simulink model "Logan"  (R2024b)
settings: Solver=ode4  StartTime=0  StopTime=inf  FixedStep=0.01  RelTol=1e-3
values from neighbouring files (symbols this model uses):
  AltPoint = 100000    [Logan_init.m]
  area_secao = 79.402*1.5    (= 119.103)    [Logan_init.m]
  b = 9    [Logan_init.m]
  c = 15.252    [Logan_init.m]
  cp = 1003    [Logan_init.m]
  E = 110e9    (= 110000000000)    [Logan_init.m]
  eta_comb = 0.95    [Logan_init.m]
  Fuel_Freeze = 0    [Logan_init.m]
  g = 9.80665    [Logan_init.m]
  gamma = 1.4    [Logan_init.m]
  GammaRef_deg = 0    [Logan_init.m]
  h1 = 0.5746    [Logan_init.m]
  h2 = 0.7752    [Logan_init.m]
  h3 = 0.1502    [Logan_init.m]
  hc = h1 + h2 + h3    (= 1.5)    [Logan_init.m]
  he = 2.6    [Logan_init.m]
  Inertia = [Ixx 0 -Ixz; 0 Iyy 0; -Ixz 0 Izz]    [Logan_init.m]
  L = 22.5    [Logan_init.m]
  L_inlet = 5.5    [Logan_init.m]
  La = 5    [Logan_init.m]
  LHV = 120 * 10^6    (= 120000000)    [Logan_init.m]
  Ln0 = 4.8    [Logan_init.m]
  MachPoint = 10    [Logan_init.m]
  Manual_Control = 0    [Logan_init.m]
  MW_air = 28.85    [Logan_init.m]
  MW_H2 = 2.00    (= 2)    [Logan_init.m]
  PA_EngineMode = 0    [Logan_init.m]
  PA_LatMode = 2    [Logan_init.m]
  PA_LongMode = 2    [Logan_init.m]
  PA_TECSEngineInput = 0    [Logan_init.m]
  PhiPoint = 0    [Logan_init.m]
  R = 287    [Logan_init.m]
  RefMass_kg = 31000    [Logan_init.m]
  S = 91.5    [Logan_init.m]
  tau1 = 3.1    [Logan_init.m]
  tau2 = 18.23    [Logan_init.m]
  TECS_ON = 0    [Logan_init.m]
  theta1 = 4    [Logan_init.m]
  theta2 = 6    [Logan_init.m]
  theta_n = 4    [Logan_init.m]
  ThetaPoint = 0    [Logan_init.m]
  Trimming = 0    [Logan_init.m]    (also in Logan_trim.m)
  w = 3.000    (= 3)    [Logan_init.m]
  Waypoint_idx = 1    [Logan_init.m]
  Waypoints = [ ... (first row only)    [Logan_init.m]
  x_a = 3.7    [Logan_init.m]
  x_inlet = 6    [Logan_init.m]
  x_n0 = 3    [Logan_init.m]
  xf_m = 0    [Logan_init.m]
  y_cg = 0    [Logan_init.m]
  z_a = 0.4    [Logan_init.m]
  z_cg = -0.996    [Logan_init.m]
  z_inlet = 0.7    [Logan_init.m]
  zf_m = 0    [Logan_init.m]
undefined symbols (not defined in the file or in its folder): Earth, Receive, Send, WGS84
libraries: simulink x4, spsFirstOrderFilterLib x4, aerolibactuator x3, aerolibfltsims x2, aerolibatmos2 x1, aerolibtransform2 x1, aerolibanimutils x1, dspswit3 x1, spsEdgeDetectorLib x1
(part 2 of 5)

== system Logan/EqM/ExtForcesMoments ==
  LBE : Inport
  Mass_kg : Inport  Port=2
  GroundForcesMoments_N_Nm : Inport  Port=3
  AeroForcesMoments_N_Nm : Inport  Port=4
  ThrustForcesMoments_N_Nm : Inport  Port=5
  Add : Sum  Inputs=+++
  Constant : Constant  Value=0
  Demux : Demux  Outputs=2
  Demux1 : Demux  Outputs=3
  Divide : Product  Inputs=*/  Multiplication=Matrix(*)
  Gain : Gain  Gain=-1
  Math Function : Math  Operator=transpose  SignedPower=on
  Mux : Mux  Inputs=3
  Mux1 : Mux  Inputs=3
  Product : Product  Multiplication=Matrix(*)
  Sum : Sum  Inputs=|++
  g_mps2 : Gain  Gain=g
  ExtForces_N : Outport
  ExtMoments_Nm : Outport  Port=2
  LoadFactors : Outport  Port=3
  wires:
  Product/1 -> Sum/1  "Weight_N_body"
  Sum/1 -> ExtForces_N/1
  Divide/1 -> Demux1/1
  ThrustForcesMoments_N_Nm/1 -> Add/3
  Mux/1 -> Product/2
  Add/1 -> Demux/1
  LBE/1 -> Math Function/1
  g_mps2/1 -> Mux/3, Divide/2  "Weight_N"
  Mass_kg/1 -> g_mps2/1
  Demux1/1 -> Mux1/1  "nx"
  Demux1/2 -> Mux1/2  "ny"
  AeroForcesMoments_N_Nm/1 -> Add/2
  Mux1/1 -> LoadFactors/1
  Demux1/3 -> Gain/1
  Gain/1 -> Mux1/3  "nz"
  Demux/2 -> ExtMoments_Nm/1  "Moments"
  Constant/1 -> Mux/1, Mux/2
  GroundForcesMoments_N_Nm/1 -> Add/1
  Math Function/1 -> Product/1  "LEB"
  Demux/1 -> Divide/1, Sum/2  "Forces"

== system Logan/EqM/InertialData ==
  VB_mps : Inport
  LBE : Inport  Port=2
  Demux : Demux  Outputs=3
  Mux : Mux  Inputs=3
  Product : Product  Multiplication=Matrix(*)
  XI_m : Integrator  ContinuousStateAttributes='XI_m'
  YI_m1 : Integrator  ContinuousStateAttributes='YI_m'
  ZI_m : Integrator  ContinuousStateAttributes='ZI_m'
  PositionIntertial_m : Outport
  InertialVelocity_mps : Outport  Port=2
  wires:
  Demux/3 -> ZI_m/1
  Demux/2 -> YI_m1/1
  Demux/1 -> XI_m/1
  Product/1 -> Demux/1, InertialVelocity_mps/1  "VI_mps"
  ZI_m/1 -> Mux/3
  XI_m/1 -> Mux/1
  YI_m1/1 -> Mux/2
  Mux/1 -> PositionIntertial_m/1
  VB_mps/1 -> Product/2
  LBE/1 -> Product/1

== system Logan/EqM/TrajectoryData ==
  VI_mps : Inport
  Add : Sum
  Demux : Demux  Outputs=3
  Gain : Gain  Gain=-1
  Gain1 : Gain  Gain=180/pi
  Gain2 : Gain  Gain=180/pi
  Math Function : Math  Operator=square  SignedPower=on
  Math Function1 : Math  Operator=square  SignedPower=on
  Sqrt : Sqrt
  Trigonometric Function : Trigonometry  Operator=atan2
  Trigonometric Function1 : Trigonometry  Operator=atan2
  GroundSpeed_mps : Outport
  Gamma_deg : Outport  Port=2
  Track_deg : Outport  Port=3
  wires:
  VI_mps/1 -> Demux/1
  Trigonometric Function1/1 -> Gain2/1
  Gain/1 -> Trigonometric Function/1
  Add/1 -> Sqrt/1
  Demux/1 -> Math Function/1, Trigonometric Function1/2
  Sqrt/1 -> Trigonometric Function/2, GroundSpeed_mps/1
  Demux/2 -> Math Function1/1, Trigonometric Function1/1
  Demux/3 -> Gain/1
  Trigonometric Function/1 -> Gain1/1
  Math Function1/1 -> Add/2
  Math Function/1 -> Add/1
  Gain1/1 -> Gamma_deg/1
  Gain2/1 -> Track_deg/1

== system Logan/Inner Loop/EngineControl ==
  MachCmd : Inport
  Mach : Inport  Port=2
  Add7 : Sum  Inputs=+++
  Derivative1 : Derivative
  Gain21 : Gain  Gain=0.4
  Gain3 : Gain  Gain=8
  Gain6 : Gain  Gain=11
  Integrator3 : Integrator  LimitOutput=on  UpperSaturationLimit=10  LowerSaturationLimit=-1  ContinuousStateAttributes='Engine_MachInt'
  Sum18 : Sum  Inputs=|+-
  EngineCmd : Outport
  wires:
  MachCmd/1 -> Sum18/1
  Derivative1/1 -> Gain6/1
  Gain3/1 -> Add7/2
  Mach/1 -> Sum18/2
  Gain6/1 -> Add7/3
  Gain21/1 -> Add7/1
  Integrator3/1 -> Gain21/1
  Add7/1 -> EngineCmd/1
  Sum18/1 -> Derivative1/1, Gain3/1, Integrator3/1

== system Logan/Inner Loop/LateroDirectionalControl ==
  PhiCmd : Inport
  p_rps : Inport  Port=2
  r_rps : Inport  Port=3
  Beta_deg : Inport  Port=4
  Phi_deg : Inport  Port=5
  Add4 : Sum  Inputs=+++
  Add5 : Sum  Inputs=+++
  Beta_ref : Constant  Value=0
  Gain : Gain  Gain=-1.2
  Gain1 : Gain  Gain=pi/180
  Gain16 : Gain  Gain=0.3
  Gain17 : Gain  Gain=0.15
  Gain2 : Gain  Gain=-0.55
  Gain4 : Gain  Gain=-0.03
  Gain5 : Gain  Gain=-0.015
  Integrator : Integrator  ContinuousStateAttributes='Lat_PhiInt'
  Integrator1 : Integrator  ContinuousStateAttributes='Lat_BetaInt'
  Sum7 : Sum  Inputs=|+-
  Sum8 : Sum  Inputs=|+-
  AileronCmd : Outport
  RudderCmd : Outport  Port=2
  wires:
  Beta_deg/1 -> Sum8/2, Gain5/1  "Beta"
  Gain16/1 -> Add5/1
  Integrator1/1 -> Gain16/1
  Add5/1 -> RudderCmd/1
  Sum7/1 -> Gain1/1
  p_rps/1 -> Gain/1
  Add4/1 -> AileronCmd/1
  Gain17/1 -> Add4/1
  Integrator/1 -> Gain17/1
  Beta_ref/1 -> Sum8/1
  Gain5/1 -> Add5/2
  Gain2/1 -> Add5/3
  Gain4/1 -> Add4/2
  PhiCmd/1 -> Sum7/1
  r_rps/1 -> Gain2/1
  Phi_deg/1 -> Sum7/2, Gain4/1
  Sum8/1 -> Integrator1/1
  Gain1/1 -> Integrator/1
  Gain/1 -> Add4/3  "p_rps"

== system Logan/Inner Loop/LongitudinalControl ==
  Gamma_deg : Inport
  AlphaDot_rps : Inport  Port=2
  Q_Dyn_Pa : Inport  Port=3
  GammaCmd : Inport  Port=4
  Add6 : Sum  Inputs=+++
  GainScheduling1 : Subsystem
  GainScheduling2 : Subsystem
  GainScheduling3 : Subsystem
  Integrator2 : Integrator  LimitOutput=on  UpperSaturationLimit=8  LowerSaturationLimit=-8  ContinuousStateAttributes='Long_GammaInt'
  Sum16 : Sum  Inputs=|+-
  ElevCmd : Outport
  wires:
  Add6/1 -> ElevCmd/1
  GammaCmd/1 -> Sum16/1
  Gamma_deg/1 -> [Gamma_deg]
  [Gamma_deg] -> Sum16/2
  Sum16/1 -> Integrator2/1
  Q_Dyn_Pa/1 -> [Q_Dyn_Pa]
  [Q_Dyn_Pa] -> GainScheduling3/2(Q_Dyn_Pa)
  [Q_Dyn_Pa] -> GainScheduling1/2(Q_Dyn_Pa)
  [Q_Dyn_Pa] -> GainScheduling2/2(Q_Dyn_Pa)
  [Gamma_deg] -> GainScheduling1/1(Gamma_deg)
  GainScheduling1/1(Out1) -> Add6/1
  GainScheduling2/1(Out1) -> Add6/2
  Integrator2/1 -> GainScheduling2/1(GammaCmd)
  GainScheduling3/1(Out1) -> Add6/3
  AlphaDot_rps/1 -> GainScheduling3/1(AlphaDot_rps)

== system Logan/Inner Loop/Trimming ==
  ElevCmd : Inport
  Constant10 : Constant  Value=Trimming
  Constant9 : Constant  Value=0
  Switch : Switch  Criteria=u2 > Threshold  Threshold=0.5  SaturateOnIntegerOverflow=off  InputSameDT=off
  DeltaElevCmd : Outport
  wires:
  Constant9/1 -> Switch/1
  Constant10/1 -> Switch/2
  Switch/1 -> DeltaElevCmd/1
  ElevCmd/1 -> Switch/3

== system Logan/Inner Loop/Trimming1 ==
  AileronCmd : Inport
  Constant10 : Constant  Value=Trimming
  Constant9 : Constant  Value=0
  Switch : Switch  Criteria=u2 > Threshold  Threshold=0.5  SaturateOnIntegerOverflow=off  InputSameDT=off
  DeltaAileronCmd : Outport
  wires:
  Constant9/1 -> Switch/1
  Constant10/1 -> Switch/2
  Switch/1 -> DeltaAileronCmd/1
  AileronCmd/1 -> Switch/3

== system Logan/Inner Loop/Trimming2 ==
  RudderCmd : Inport
  Constant10 : Constant  Value=Trimming
  Constant9 : Constant  Value=0
  Switch : Switch  Criteria=u2 > Threshold  Threshold=0.5  SaturateOnIntegerOverflow=off  InputSameDT=off
  DeltaRudderCmd : Outport
  wires:
  Constant9/1 -> Switch/1
  Constant10/1 -> Switch/2
  Switch/1 -> DeltaRudderCmd/1
  RudderCmd/1 -> Switch/3

== system Logan/Inner Loop/Trimming3 ==
  EngineCmd : Inport
  Constant10 : Constant  Value=Trimming
  Constant9 : Constant  Value=0
  Switch : Switch  Criteria=u2 > Threshold  Threshold=0.5  SaturateOnIntegerOverflow=off  InputSameDT=off
  DeltaEngineCmd : Outport
  wires:
  Constant9/1 -> Switch/1
  Constant10/1 -> Switch/2
  Switch/1 -> DeltaEngineCmd/1
  EngineCmd/1 -> Switch/3

== system Logan/Mass Consumption/Fuel_Freeze ==
  1 : Inport
  Constant : Constant  Value=Fuel_Freeze
  Constant17 : Constant  Value=0
  Constant8 : Constant  Value=Trimming
  Logical Operator : Logic  Operator=OR  AllPortsSameDT=off  OutDataTypeStr=boolean
  Switch6 : Switch  Criteria=u2 > Threshold  Threshold=0.5  SaturateOnIntegerOverflow=off  InputSameDT=off
  2 : Outport
  wires:
  Constant17/1 -> Switch6/1
  1/1 -> Switch6/3
  Switch6/1 -> 2/1
  Logical Operator/1 -> Switch6/2
  Constant8/1 -> Logical Operator/1
  Constant/1 -> Logical Operator/2

== system Logan/Outer Loop/AltitudeMode ==
  Alt_ft : Inport
  Add8 : Sum
  AltPoint : Constant  Value=AltPoint
  Derivative2 : Derivative
  First-Order Filter3 : spsFirstOrderFilterLib/First-Order Filter  FilterType=Lowpass  Tc=0.5  Ts=0  Initialize=off  Vac_Init=[0, 0, 60]  Vdc_Init=0  PlotResponse=off  FreqRange="[0,  200,  1]"
  Gain11 : Gain  Gain=64e-5
  Gain12 : Gain  Gain=-128e-5
  Saturation7 : Saturate  UpperLimit=3  LowerLimit=-3
  Sum14 : Sum  Inputs=|+-
  Trimming1 : Subsystem
  AltRef : Outport
  wires:
  Gain12/1 -> Add8/2
  Alt_ft/1 -> Sum14/2, Derivative2/1
  Derivative2/1 -> Gain12/1
  Add8/1 -> Saturation7/1
  AltPoint/1 -> Sum14/1
  First-Order Filter3/1 -> Add8/1
  Sum14/1 -> Gain11/1
  Saturation7/1 -> AltRef/1
  Gain11/1 -> Trimming1/1(1)
  Trimming1/1(2) -> First-Order Filter3/1

== system Logan/Outer Loop/BankMode ==
  Phi_deg : Inport
  p_rps : Inport  Port=2
  Add8 : Sum  Inputs=+++
  Gain : Gain  Gain=1.2
  Gain11 : Gain  Gain=0.4
  Gain12 : Gain  Gain=1.2
  Integrator : Integrator
  PhiPoint : Constant  Value=PhiPoint
  Saturation : Saturate  UpperLimit=45  LowerLimit=-45
  Sum14 : Sum  Inputs=|+-
  Trimming1 : Subsystem
  PhiRef : Outport
  wires:
  Phi_deg/1 -> Sum14/2
  Add8/1 -> Saturation/1
  PhiPoint/1 -> Sum14/1
  Gain11/1 -> Add8/1
  p_rps/1 -> Gain12/1
  Saturation/1 -> PhiRef/1
  Sum14/1 -> Trimming1/1(1), Gain/1
  Integrator/1 -> Gain11/1
  Gain12/1 -> Add8/3
  Gain/1 -> Add8/2
  Trimming1/1(2) -> Integrator/1

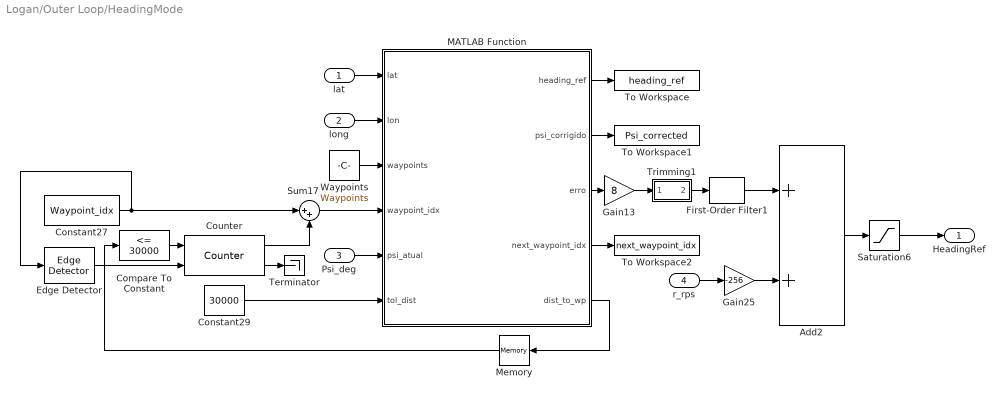
== system Logan/Outer Loop/HeadingMode ==
  lat : Inport
  long : Inport  Port=2
  Psi_deg : Inport  Port=3
  r_rps : Inport  Port=4
  Add2 : Sum
  Compare To Constant : simulink/Logic and Bit Operations/Compare To Constant  relop=<=  const=30000  OutDataTypeStr=boolean
  Constant27 : Constant  Value=Waypoint_idx  OutDataTypeStr=double
  Constant29 : Constant  Value=30000
  Counter : dspswit3/Counter  Direction=Up  CountEvent=Rising edge  CounterSize=User defined  MaxCount=255  InitialCount=0  Output=Count and Hit  HitValue=32  ResetInput=on  SamplesPerFrame=1  Ts=1  CntDtype=double  HitDtype=Logical
  Edge Detector : spsEdgeDetectorLib/Edge Detector  model=Either  ic=0  Ts=0
      settings: LibrarySourceBlock=sps_lib/Control/Edge Detector
  First-Order Filter1 : spsFirstOrderFilterLib/First-Order Filter  FilterType=Lowpass  Tc=10  Ts=0  Initialize=off  Vac_Init=[0, 0, 60]  Vdc_Init=0  PlotResponse=off  FreqRange="[0,  200,  1]"
  Gain13 : Gain  Gain=8
  Gain25 : Gain  Gain=-256
  MATLAB Function : MATLAB Function  TreatAsAtomicUnit=on
  Memory : Memory
  Saturation6 : Saturate  UpperLimit=75  LowerLimit=-75
  Sum17 : Sum  Inputs=|++
  Terminator : Terminator
  To Workspace : ToWorkspace  VariableName=heading_ref  SampleTime=-1
      settings: Save2DSignal=2-D array (concatenate along first dimension)
  To Workspace1 : ToWorkspace  VariableName=Psi_corrected  SampleTime=-1
      settings: Save2DSignal=2-D array (concatenate along first dimension)
  To Workspace2 : ToWorkspace  VariableName=next_waypoint_idx  SampleTime=-1
      settings: Save2DSignal=2-D array (concatenate along first dimension)
  Trimming1 : Subsystem
  Waypoints : Constant  Value=Waypoints  VectorParams1D=off
  HeadingRef : Outport
  wires:
  MATLAB Function/3(erro) -> Gain13/1
  MATLAB Function/4(next_waypoint_idx) -> To Workspace2/1
  Constant27/1 -> Edge Detector/1, Sum17/1
  Compare To Constant/1 -> Counter/1
  MATLAB Function/1(heading_ref) -> To Workspace/1
  Saturation6/1 -> HeadingRef/1
  Edge Detector/1 -> Counter/2
  Psi_deg/1 -> MATLAB Function/5(psi_atual)
  MATLAB Function/5(dist_to_wp) -> Memory/1
  long/1 -> MATLAB Function/2(lon)
  Sum17/1 -> MATLAB Function/4(waypoint_idx)
  MATLAB Function/2(psi_corrigido) -> To Workspace1/1
  Counter/2 -> Terminator/1
  Counter/1 -> Sum17/2
  Constant29/1 -> MATLAB Function/6(tol_dist)
  Memory/1 -> Compare To Constant/1
  lat/1 -> MATLAB Function/1(lat)
  First-Order Filter1/1 -> Add2/1
  Waypoints/1 -> MATLAB Function/3(waypoints)
  Gain25/1 -> Add2/2
  r_rps/1 -> Gain25/1
  Add2/1 -> Saturation6/1
  Gain13/1 -> Trimming1/1(1)
  Trimming1/1(2) -> First-Order Filter1/1

== system Logan/Outer Loop/MachMode ==
  MachPoint : Constant  Value=MachPoint
  Saturation : Saturate  UpperLimit=10  LowerLimit=5
  MachRef : Outport
  wires:
  MachPoint/1 -> Saturation/1
  Saturation/1 -> MachRef/1

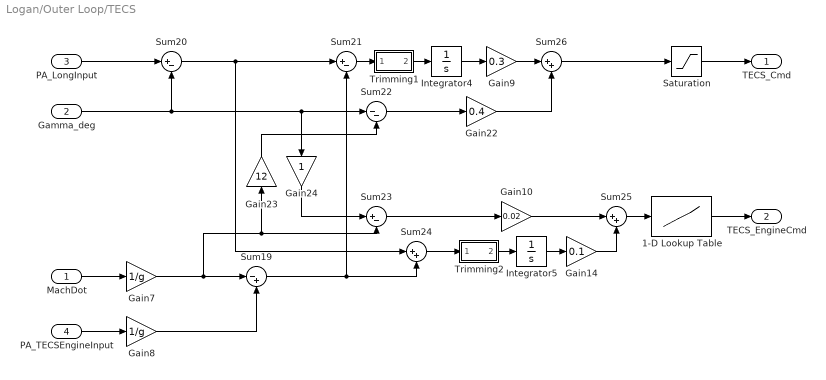
== system Logan/Outer Loop/TECS ==
  MachDot : Inport
  Gamma_deg : Inport  Port=2
  PA_LongInput : Inport  Port=3
  PA_TECSEngineInput : Inport  Port=4
  1-D Lookup Table : Lookup_n-D  NumberOfTableDimensions=1  BreakpointsForDimension1=[-5;-4;-3;-2;-1;0;1;2;3;4;5]  Table=[-1;-0.80000000000000004;-0.59999999999999998;-0.40000000000000002;-0.20000000000000001;0;0.20000000000000001;0.40000000000000002;0.59999999999999998;0.80000000000000004;1]  InternalRulePriority=Speed  RndMeth=Simplest
  Gain10 : Gain  Gain=0.02
  Gain14 : Gain  Gain=0.1
  Gain22 : Gain  Gain=0.4
  Gain23 : Gain  Gain=12
  Gain24 : Gain
  Gain7 : Gain  Gain=1/g
  Gain8 : Gain  Gain=1/g
  Gain9 : Gain  Gain=0.3
  Integrator4 : Integrator  UpperSaturationLimit=10  LowerSaturationLimit=-10
  Integrator5 : Integrator
  Saturation : Saturate  UpperLimit=3  LowerLimit=-3
  Sum19 : Sum  Inputs=|-+
  Sum20 : Sum  Inputs=|+-
  Sum21 : Sum  Inputs=|+-
  Sum22 : Sum  Inputs=|--
  Sum23 : Sum  Inputs=|+-
  Sum24 : Sum  Inputs=|++
  Sum25 : Sum  Inputs=|++
  Sum26 : Sum  Inputs=|++
  Trimming1 : Subsystem
  Trimming2 : Subsystem
  TECS_Cmd : Outport
  TECS_EngineCmd : Outport  Port=2
  wires:
  1-D Lookup Table/1 -> TECS_EngineCmd/1
  Sum23/1 -> Gain10/1
  Gamma_deg/1 -> Sum22/1, Gain24/1, Sum20/2
  Sum19/1 -> Sum21/2, Sum24/2
  Gain22/1 -> Sum26/2
  Sum22/1 -> Gain22/1
  PA_TECSEngineInput/1 -> Gain8/1
  Sum20/1 -> Sum21/1, Sum24/1
  Sum25/1 -> 1-D Lookup Table/1
  Gain7/1 -> Sum23/2, Gain23/1, Sum19/1
  Sum24/1 -> Trimming2/1(1)
  Gain23/1 -> Sum22/2
  Gain8/1 -> Sum19/2
  Gain10/1 -> Sum25/1
  Integrator5/1 -> Gain14/1
  Gain24/1 -> Sum23/1
  Integrator4/1 -> Gain9/1
  Gain9/1 -> Sum26/1
  Gain14/1 -> Sum25/2
  MachDot/1 -> Gain7/1
  PA_LongInput/1 -> Sum20/1
  Sum21/1 -> Trimming1/1(1)
  Trimming1/1(2) -> Integrator4/1
  Trimming2/1(2) -> Integrator5/1
  Sum26/1 -> Saturation/1
  Saturation/1 -> TECS_Cmd/1

== system Logan/Outer Loop/ThetaMode ==
  Theta_deg : Inport
  q_rps : Inport  Port=2
  Add8 : Sum  Inputs=+++
  Gain : Gain  Gain=1.4
  Gain11 : Gain  Gain=0.4
  Gain12 : Gain  Gain=0.6
  Integrator : Integrator
  Saturation : Saturate  UpperLimit=10  LowerLimit=-10
  Sum14 : Sum  Inputs=|+-
  ThetaPoint : Constant  Value=ThetaPoint
  Trimming1 : Subsystem
  ThetaRef : Outport
  wires:
  Theta_deg/1 -> Sum14/2
  Add8/1 -> Saturation/1
  ThetaPoint/1 -> Sum14/1
  q_rps/1 -> Gain12/1
  Gain11/1 -> Add8/1
  Saturation/1 -> ThetaRef/1
  Integrator/1 -> Gain11/1
  Gain12/1 -> Add8/3
  Gain/1 -> Add8/2
  Sum14/1 -> Trimming1/1(1)
  Trimming1/1(2) -> Gain/1, Integrator/1

== system Logan/Outer Loop/Trimming ==
  HeadingRef : Inport
  Constant22 : Constant  Value=0
  Constant23 : Constant  Value=Trimming
  Switch7 : Switch  Criteria=u2 > Threshold  Threshold=0.5  SaturateOnIntegerOverflow=off  InputSameDT=off
  PA_HeadingRef : Outport
  wires:
  Constant23/1 -> Switch7/2
  Constant22/1 -> Switch7/1
  Switch7/1 -> PA_HeadingRef/1
  HeadingRef/1 -> Switch7/3

== system Logan/Outer Loop/Trimming1 ==
  ThetaRef : Inport
  Constant17 : Constant  Value=0
  Constant8 : Constant  Value=Trimming
  Switch6 : Switch  Criteria=u2 > Threshold  Threshold=0.5  SaturateOnIntegerOverflow=off  InputSameDT=off
  PA_ThetaRef : Outport
  wires:
  Constant8/1 -> Switch6/2
  Constant17/1 -> Switch6/1
  ThetaRef/1 -> Switch6/3
  Switch6/1 -> PA_ThetaRef/1

== system Logan/Outer Loop/Trimming2 ==
  AltRef : Inport
  Constant17 : Constant  Value=0
  Constant8 : Constant  Value=Trimming
  Switch6 : Switch  Criteria=u2 > Threshold  Threshold=0.5  SaturateOnIntegerOverflow=off  InputSameDT=off
  PA_AltRef : Outport
  wires:
  Constant8/1 -> Switch6/2
  Constant17/1 -> Switch6/1
  AltRef/1 -> Switch6/3
  Switch6/1 -> PA_AltRef/1

== system Logan/Outer Loop/Trimming3 ==
  PhiRef : Inport
  Constant17 : Constant  Value=0
  Constant8 : Constant  Value=Trimming
  Switch6 : Switch  Criteria=u2 > Threshold  Threshold=0.5  SaturateOnIntegerOverflow=off  InputSameDT=off
  PA_PhiRef : Outport
  wires:
  Constant8/1 -> Switch6/2
  Constant17/1 -> Switch6/1
  PhiRef/1 -> Switch6/3
  Switch6/1 -> PA_PhiRef/1

== system Logan/Outer Loop/Trimming4 ==
  MachRef : Inport
  Constant17 : Constant  Value=0
  Constant8 : Constant  Value=Trimming
  Switch6 : Switch  Criteria=u2 > Threshold  Threshold=0.5  SaturateOnIntegerOverflow=off  InputSameDT=off
  PA_EngineCmd : Outport
  wires:
  Constant8/1 -> Switch6/2
  Constant17/1 -> Switch6/1
  MachRef/1 -> Switch6/3
  Switch6/1 -> PA_EngineCmd/1

== system Logan/Outer Loop/Trimming5 ==
  TECS : Inport
  Constant17 : Constant  Value=0
  Constant8 : Constant  Value=Trimming
  Switch6 : Switch  Criteria=u2 > Threshold  Threshold=0.5  SaturateOnIntegerOverflow=off  InputSameDT=off
  TECS_EngineCmd : Outport
  wires:
  Constant8/1 -> Switch6/2
  Constant17/1 -> Switch6/1
  TECS/1 -> Switch6/3
  Switch6/1 -> TECS_EngineCmd/1

== system Logan/Outer Loop/Trimming6 ==
  TECS : Inport
  Constant17 : Constant  Value=0
  Constant8 : Constant  Value=Trimming
  Switch6 : Switch  Criteria=u2 > Threshold  Threshold=0.5  SaturateOnIntegerOverflow=off  InputSameDT=off
  TECS_Cmd : Outport
  wires:
  Constant8/1 -> Switch6/2
  Constant17/1 -> Switch6/1
  TECS/1 -> Switch6/3
  Switch6/1 -> TECS_Cmd/1

== system Logan/Propulsion/EngineDynamics ==
  Thrust : Inport
  Filter_init : Subsystem
  First-Order Filter : spsFirstOrderFilterLib/First-Order Filter  FilterType=Lowpass  Tc=0.5  Ts=0  Initialize=off  Vac_Init=[0, 0, 60]  Vdc_Init=0  PlotResponse=off  FreqRange="[0,  200,  1]"
  Trimming : Subsystem
  T_thrust : Outport
  wires:
  Thrust/1 -> Trimming/2(Thrust), Filter_init/1(1)
  Trimming/1(T_Thrust) -> T_thrust/1
  First-Order Filter/1 -> Trimming/1(Thrust_Dyn)
  Filter_init/1(2) -> First-Order Filter/1

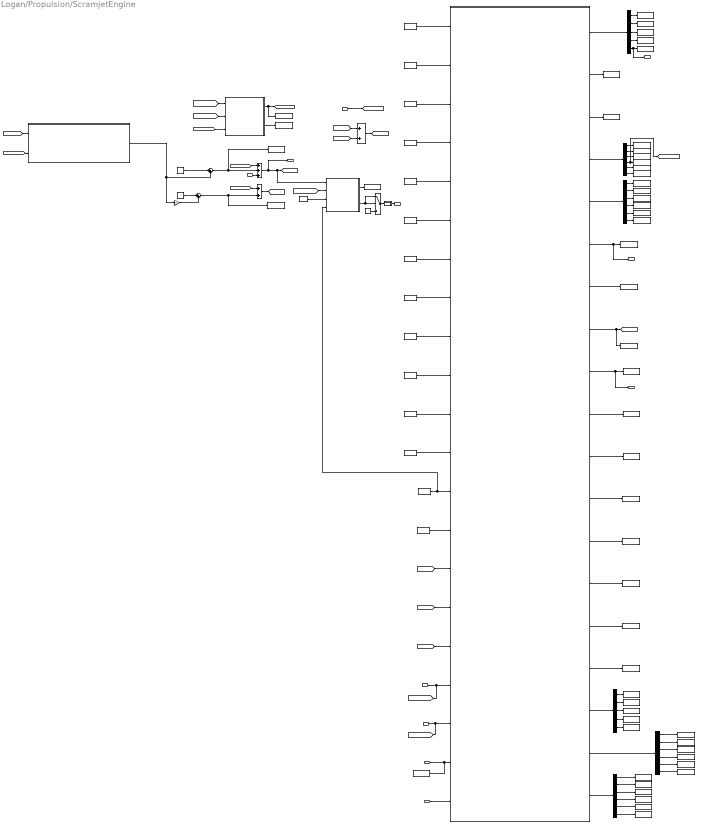
== system Logan/Propulsion/ScramjetEngine ==
  M1 : Inport
  T1 : Inport  Port=2
  p1 : Inport  Port=3
  Alpha : Inport  Port=4
  throttle : Inport  Port=5
  Delta_tau_f : Inport  Port=6
  Add : Sum  Inputs=+++
  Add1 : Sum
  Add2 : Sum
  Constant : Constant  Value=theta1
  Constant1 : Constant  Value=theta2
  Constant10 : Constant  Value=w
  Constant11 : Constant  Value=h1
  Constant12 : Constant  Value=h2
  Constant13 : Constant  Value=h3
  Constant14 : Constant  Value=hc
  Constant15 : Constant  Value=he
  Constant16 : Constant  Value=L_inlet
  Constant17 : Constant  Value=0
  Constant2 : Constant  Value=R
  Constant3 : Constant  Value=gamma
  Constant4 : Constant  Value=g
  Constant5 : Constant  Value=MW_H2
  Constant6 : Constant  Value=MW_air
  Constant7 : Constant  Value=LHV
  Constant8 : Constant  Value=eta_comb
  Constant9 : Constant  Value=cp
  Demux{,1,4..5} (4 alike) : Demux  Outputs=6
  Demux2 : Demux  Outputs=5
  Demux3 : Demux  Outputs=5
  Gain3 : Gain  Gain=2
  Ramp_Control : Subsystem
  Sum : Sum  Inputs=|++
  Sum1 : Sum  Inputs=|++
  Switch : Switch  Criteria=u2 > Threshold  SaturateOnIntegerOverflow=off  InputSameDT=off
  ThermodynamicModel : MATLAB Function  TreatAsAtomicUnit=on
  To Workspace : ToWorkspace  VariableName=m_dot_fuel  SampleTime=-1
      settings: Save2DSignal=2-D array (concatenate along first dimension)
  To Workspace1 : ToWorkspace  VariableName=M_ign  SampleTime=-1
      settings: Save2DSignal=2-D array (concatenate along first dimension)
  To Workspace10 : ToWorkspace  VariableName=M5  SampleTime=-1
      settings: Save2DSignal=2-D array (concatenate along first dimension)
  To Workspace11 : ToWorkspace  VariableName=M6  SampleTime=-1
      settings: Save2DSignal=2-D array (concatenate along first dimension)
  To Workspace12 : ToWorkspace  VariableName=M3  SampleTime=-1
      settings: Save2DSignal=2-D array (concatenate along first dimension)
  To Workspace13 : ToWorkspace  VariableName=ShockPoint  SampleTime=-1
      settings: Save2DSignal=2-D array (concatenate along first dimension)
  To Workspace14 : ToWorkspace  VariableName=T_ign  SampleTime=-1
      settings: Save2DSignal=2-D array (concatenate along first dimension)
  To Workspace15 : ToWorkspace  VariableName=p2  SampleTime=-1
      settings: Save2DSignal=2-D array (concatenate along first dimension)
  To Workspace16 : ToWorkspace  VariableName=p01  SampleTime=-1
      settings: Save2DSignal=2-D array (concatenate along first dimension)
  To Workspace17 : ToWorkspace  VariableName=T0  SampleTime=-1
      settings: Save2DSignal=2-D array (concatenate along first dimension)
  To Workspace18 : ToWorkspace  VariableName=p3  SampleTime=-1
      settings: Save2DSignal=2-D array (concatenate along first dimension)
  To Workspace19 : ToWorkspace  VariableName=p4  SampleTime=-1
      settings: Save2DSignal=2-D array (concatenate along first dimension)
  To Workspace2 : ToWorkspace  VariableName=T05_T0star_ratio  SampleTime=-1
      settings: Save2DSignal=2-D array (concatenate along first dimension)
  To Workspace20 : ToWorkspace  VariableName=p5  SampleTime=-1
      settings: Save2DSignal=2-D array (concatenate along first dimension)
  To Workspace21 : ToWorkspace  VariableName=p6  SampleTime=-1
      settings: Save2DSignal=2-D array (concatenate along first dimension)
  To Workspace22 : ToWorkspace  VariableName=T1  SampleTime=-1
      settings: Save2DSignal=2-D array (concatenate along first dimension)
  To Workspace23 : ToWorkspace  VariableName=fuel_air_ratio  SampleTime=-1
      settings: Save2DSignal=2-D array (concatenate along first dimension)
  To Workspace24 : ToWorkspace  VariableName=T2  SampleTime=-1
      settings: Save2DSignal=2-D array (concatenate along first dimension)
  To Workspace25 : ToWorkspace  VariableName=T3  SampleTime=-1
      settings: Save2DSignal=2-D array (concatenate along first dimension)
  To Workspace26 : ToWorkspace  VariableName=T4  SampleTime=-1
      settings: Save2DSignal=2-D array (concatenate along first dimension)
  To Workspace27 : ToWorkspace  VariableName=T5  SampleTime=-1
      settings: Save2DSignal=2-D array (concatenate along first dimension)
  To Workspace28 : ToWorkspace  VariableName=T6  SampleTime=-1
      settings: Save2DSignal=2-D array (concatenate along first dimension)
  To Workspace29 : ToWorkspace  VariableName=T_thrust  SampleTime=-1
      settings: Save2DSignal=2-D array (concatenate along first dimension)
  To Workspace3 : ToWorkspace  VariableName=q  SampleTime=-1
      settings: Save2DSignal=2-D array (concatenate along first dimension)
  To Workspace30 : ToWorkspace  VariableName=theta1_deg  SampleTime=-1
      settings: Save2DSignal=2-D array (concatenate along first dimension)
  To Workspace31 : ToWorkspace  VariableName=theta2_deg  SampleTime=-1
      settings: Save2DSignal=2-D array (concatenate along first dimension)
  To Workspace32 : ToWorkspace  VariableName=p1  SampleTime=-1
      settings: Save2DSignal=2-D array (concatenate along first dimension)
  To Workspace33 : ToWorkspace  VariableName=eta_t  SampleTime=-1
      settings: Save2DSignal=2-D array (concatenate along first dimension)
  To Workspace34 : ToWorkspace  VariableName=eta_prop  SampleTime=-1
      settings: Save2DSignal=2-D array (concatenate along first dimension)
  To Workspace35 : ToWorkspace  VariableName=q1  SampleTime=-1
      settings: Save2DSignal=2-D array (concatenate along first dimension)
  To Workspace36 : ToWorkspace  VariableName=eta_ex  SampleTime=-1
      settings: Save2DSignal=2-D array (concatenate along first dimension)
  To Workspace37 : ToWorkspace  VariableName=q2  SampleTime=-1
      settings: Save2DSignal=2-D array (concatenate along first dimension)
  To Workspace38 : ToWorkspace  VariableName=q3  SampleTime=-1
      settings: Save2DSignal=2-D array (concatenate along first dimension)
  To Workspace39 : ToWorkspace  VariableName=q4  SampleTime=-1
      settings: Save2DSignal=2-D array (concatenate along first dimension)
  To Workspace4 : ToWorkspace  VariableName=Inlet_drag  SampleTime=-1
      settings: Save2DSignal=2-D array (concatenate along first dimension)
  To Workspace40 : ToWorkspace  VariableName=q5  SampleTime=-1
      settings: Save2DSignal=2-D array (concatenate along first dimension)
  To Workspace41 : ToWorkspace  VariableName=eta_ex2  SampleTime=-1
      settings: Save2DSignal=2-D array (concatenate along first dimension)
  To Workspace42 : ToWorkspace  VariableName=eta_ex3  SampleTime=-1
      settings: Save2DSignal=2-D array (concatenate along first dimension)
  To Workspace43 : ToWorkspace  VariableName=eta_ex4  SampleTime=-1
      settings: Save2DSignal=2-D array (concatenate along first dimension)
  To Workspace44 : ToWorkspace  VariableName=eta_ex1  SampleTime=-1
      settings: Save2DSignal=2-D array (concatenate along first dimension)
  To Workspace45 : ToWorkspace  VariableName=eta_ex5  SampleTime=-1
      settings: Save2DSignal=2-D array (concatenate along first dimension)
  To Workspace46 : ToWorkspace  VariableName=eta_ex_total  SampleTime=-1
      settings: Save2DSignal=2-D array (concatenate along first dimension)
  To Workspace47 : ToWorkspace  VariableName=irre_total  SampleTime=-1
      settings: Save2DSignal=2-D array (concatenate along first dimension)
  To Workspace48 : ToWorkspace  VariableName=irre_stage2  SampleTime=-1
      settings: Save2DSignal=2-D array (concatenate along first dimension)
  To Workspace49 : ToWorkspace  VariableName=irre_stage3  SampleTime=-1
      settings: Save2DSignal=2-D array (concatenate along first dimension)
  To Workspace5 : ToWorkspace  VariableName=m_dot_air  SampleTime=-1
      settings: Save2DSignal=2-D array (concatenate along first dimension)
  To Workspace50 : ToWorkspace  VariableName=irre_stage1  SampleTime=-1
      settings: Save2DSignal=2-D array (concatenate along first dimension)
  To Workspace51 : ToWorkspace  VariableName=irre_stage4  SampleTime=-1
      settings: Save2DSignal=2-D array (concatenate along first dimension)
  To Workspace52 : ToWorkspace  VariableName=irre_stage5  SampleTime=-1
      settings: Save2DSignal=2-D array (concatenate along first dimension)
  To Workspace6 : ToWorkspace  VariableName=Isp  SampleTime=-1
      settings: Save2DSignal=2-D array (concatenate along first dimension)
  To Workspace7 : ToWorkspace  VariableName=M1  SampleTime=-1
      settings: Save2DSignal=2-D array (concatenate along first dimension)
  To Workspace8 : ToWorkspace  VariableName=M2  SampleTime=-1
      settings: Save2DSignal=2-D array (concatenate along first dimension)
  To Workspace9 : ToWorkspace  VariableName=M4  SampleTime=-1
      settings: Save2DSignal=2-D array (concatenate along first dimension)
  Trimming1 : Subsystem
  calculate_T3_M3 : MATLAB Function  TreatAsAtomicUnit=on
  calculate_shock_and_door : MATLAB Function  TreatAsAtomicUnit=on
  T_thrust : Outport
  p6 : Outport  Port=2
  door_length : Outport  Port=3
  m_dot_fuel : Outport  Port=4
  theta1_deg : Outport  Port=5
  wires:
  Add/1 -> theta1_deg/1, calculate_shock_and_door/1(theta1), [theta1_deg]
  Delta_tau_f/1 -> [delta_tau_f]
  [delta_tau_f] -> Add1/1
  ThermodynamicModel/6(T_thrust) -> To Workspace29/1, T_thrust/1
  Add1/1 -> [theta2_deg]
  [theta3_deg] -> ThermodynamicModel/17(theta3)
  Alpha/1 -> Add/3
  throttle/1 -> ThermodynamicModel/21(throttle)
  [theta1_deg] -> ThermodynamicModel/15(theta1)
  [theta2_deg] -> ThermodynamicModel/16(theta2)
  [delta_tau_f] -> Add/1
  [M1] -> calculate_T3_M3/2(M1)
  [T1] -> calculate_T3_M3/1(T1)
  ThermodynamicModel/8(f) -> To Workspace23/1, [f]
  [f] -> calculate_T3_M3/3(f)
  calculate_T3_M3/1(T3) -> To Workspace14/1, [T_ign]
  calculate_T3_M3/2(M3) -> To Workspace1/1
  ThermodynamicModel/4(temperatures) -> Demux/1
  ThermodynamicModel/5(mach_numbers) -> Demux1/1
  Demux/1 -> To Workspace22/1
  Demux/2 -> To Workspace24/1
  Demux/3 -> To Workspace25/1
  Demux/5 -> To Workspace27/1
  Demux/6 -> To Workspace28/1
  Demux1/1 -> To Workspace7/1
  Demux1/2 -> To Workspace8/1
  Demux1/3 -> To Workspace12/1
  Demux1/5 -> To Workspace10/1
  Demux1/6 -> To Workspace11/1
  Add2/1 -> [theta3_deg]
  [theta1_deg] -> Add2/1
  [theta2_deg] -> Add2/2
  Constant/1 -> Sum/1
  Constant1/1 -> Sum1/1
  [T_ign] -> Ramp_Control/1(T_Ign)
  [T4] -> Ramp_Control/2(T4)
  ThermodynamicModel/1(pressures) -> Demux2/1
  Demux2/1 -> To Workspace15/1
  Demux2/2 -> To Workspace18/1
  Demux2/5 -> To Workspace21/1, p6/1
  Demux2/4 -> To Workspace20/1
  Demux2/3 -> To Workspace19/1
  Sum1/1 -> Add1/2, To Workspace31/1
  Sum/1 -> To Workspace30/1, Add/2
  Gain3/1 -> Sum1/2
  ThermodynamicModel/9(m_dot_fuel) -> To Workspace/1, m_dot_fuel/1
  Constant2/1 -> ThermodynamicModel/1(R)
  Constant3/1 -> ThermodynamicModel/2(gamma)
  Constant4/1 -> ThermodynamicModel/3(g)
  Constant5/1 -> ThermodynamicModel/4(MW_H2)
  Constant6/1 -> ThermodynamicModel/5(MW_air)
  Constant7/1 -> ThermodynamicModel/6(LHV)
  Constant8/1 -> ThermodynamicModel/7(eta_comb)
  Constant9/1 -> ThermodynamicModel/8(cp)
  Constant10/1 -> ThermodynamicModel/9(w)
  Constant11/1 -> ThermodynamicModel/10(h1)
  Constant12/1 -> ThermodynamicModel/11(h2)
  Constant13/1 -> ThermodynamicModel/12(h3)
  Constant15/1 -> ThermodynamicModel/14(he)
  ThermodynamicModel/13(T05_T0star_ratio) -> To Workspace2/1
  ThermodynamicModel/12(q) -> To Workspace3/1
  ThermodynamicModel/11(D) -> To Workspace4/1
  ThermodynamicModel/10(m_dot_air) -> To Workspace5/1
  ThermodynamicModel/7(ISP) -> To Workspace6/1
  Demux1/4 -> To Workspace9/1
  [M1] -> calculate_shock_and_door/2(Mach)
  Constant16/1 -> calculate_shock_and_door/3(L_inlet)
  calculate_shock_and_door/1(ShockPoint) -> To Workspace13/1
  ThermodynamicModel/2(p01) -> To Workspace16/1
  ThermodynamicModel/3(T0) -> To Workspace17/1
  Demux/4 -> [T4], To Workspace26/1
  Switch/1 -> Trimming1/1(1)
  calculate_shock_and_door/2(door_length) -> Switch/1, Switch/2
  Constant17/1 -> Switch/3
  Trimming1/1(2) -> door_length/1
  Ramp_Control/1(DeltaTheta) -> Sum/2, Gain3/1
  ThermodynamicModel/14(eta_t) -> To Workspace33/1
  ThermodynamicModel/15(eta_prop) -> To Workspace34/1
  ThermodynamicModel/16(eta_ex) -> To Workspace36/1
  Demux3/4 -> To Workspace39/1
  Demux3/3 -> To Workspace38/1
  Demux3/1 -> To Workspace35/1
  Demux3/2 -> To Workspace37/1
  Demux3/5 -> To Workspace40/1
  ThermodynamicModel/17(Heat) -> Demux3/1
  Demux4/5 -> To Workspace45/1
  Demux4/3 -> To Workspace42/1
  Demux4/4 -> To Workspace43/1
  Demux4/2 -> To Workspace41/1
  Demux4/1 -> To Workspace44/1
  ThermodynamicModel/19(eta_stages) -> Demux4/1
  Demux4/6 -> To Workspace46/1
  Demux5/5 -> To Workspace52/1
  Demux5/6 -> To Workspace47/1
  Demux5/4 -> To Workspace51/1
  Demux5/3 -> To Workspace49/1
  Demux5/2 -> To Workspace48/1
  ThermodynamicModel/18(Irre) -> Demux5/1
  Demux5/1 -> To Workspace50/1
  p1/1 -> To Workspace32/1, ThermodynamicModel/20(p1)
  Constant14/1 -> calculate_shock_and_door/4(hc), ThermodynamicModel/13(hc)
  T1/1 -> [T1], ThermodynamicModel/19(T1)
  M1/1 -> [M1], ThermodynamicModel/18(M1)

== system Logan/EqM/BodyRates/CrossProduct ==
  A : Inport
  B : Inport  Port=2
  Add : Sum  Inputs=+-
  Demux : Demux  Outputs=3
  Demux1 : Demux  Outputs=3
  Mux : Mux  Inputs=3
  Mux1 : Mux  Inputs=3
  Product{,1..5} (6 alike) : Product
  C : Outport
  wires:
  Add/1 -> C/1  "A X B"
  Product2/1 -> Mux/3
  Product/1 -> Mux/1
  Demux/1 -> Product2/1, Product4/1
  Demux1/2 -> Product2/2, Product3/2
  Demux/3 -> Product1/1, Product3/1
  B/1 -> Demux1/1
  Mux1/1 -> Add/2
  Demux/2 -> Product/1, Product5/1
  A/1 -> Demux/1
  Product3/1 -> Mux1/1
  Demux1/1 -> Product1/2, Product5/2
  Mux/1 -> Add/1
  Product5/1 -> Mux1/3
  Product1/1 -> Mux/2
  Demux1/3 -> Product/2, Product4/2
  Product4/1 -> Mux1/2

== system Logan/EqM/BodyVelocities/CrossProduct ==
  A : Inport
  B : Inport  Port=2
  Add : Sum  Inputs=+-
  Demux : Demux  Outputs=3
  Demux1 : Demux  Outputs=3
  Mux : Mux  Inputs=3
  Mux1 : Mux  Inputs=3
  Product{,1..5} (6 alike) : Product
  C : Outport
  wires:
  Add/1 -> C/1  "A X B"
  Product2/1 -> Mux/3
  Product/1 -> Mux/1
  Demux/1 -> Product2/1, Product4/1
  Demux1/2 -> Product2/2, Product3/2
  Demux/3 -> Product1/1, Product3/1
  B/1 -> Demux1/1
  Mux1/1 -> Add/2
  Demux/2 -> Product/1, Product5/1
  A/1 -> Demux/1
  Product3/1 -> Mux1/1
  Demux1/1 -> Product1/2, Product5/2
  Mux/1 -> Add/1
  Product5/1 -> Mux1/3
  Product1/1 -> Mux/2
  Demux1/3 -> Product/2, Product4/2
  Product4/1 -> Mux1/2

== system Logan/EqM/EulerAngles/EulerRates ==
  BodyRates_radps : Inport
  EulerAngles_rad : Inport  Port=2
  Abs : Abs  SaturateOnIntegerOverflow=off
  Constant : Constant  Value=0.001
  Demux : Demux  Outputs=3
  Mux : Mux  Inputs=3
  Mux1 : Mux  Inputs=3
  Mux2 : Mux  Inputs=3
  Product : Product
  Relay : Relay  OnSwitchValue=.001  OffSwitchValue=0  OnOutputValue=0  OffOutputValue=1
  Sign : Signum
  Switch : Switch  Criteria=u2 > Threshold  Threshold=0.5  SaturateOnIntegerOverflow=off  InputSameDT=off
  Trigonometric Function : Trigonometry  Operator=sincos
  phidot_radps2 : Fcn  Expr=u(1)+u(2)*u(4)*(u(5)/u(8))+u(3)*u(7)*(u(5)/u(8))
  psidot_radps2 : Fcn  Expr=(u(2)*u(4)+u(3)*u(7))/u(8)
  thetadot_radps2 : Fcn  Expr=u(2)*u(7)-u(3)*u(4)
  EulerRates_radsps2 : Outport
  wires:
  Mux1/1 -> Mux/3
  Trigonometric Function/1 -> Mux/2
  Demux/3 -> Mux1/3
  Constant/1 -> Product/1
  Sign/1 -> Product/2
  Switch/1 -> Mux1/2
  Demux/2 -> Switch/3, Abs/1, Sign/1
  Mux2/1 -> EulerRates_radsps2/1
  psidot_radps2/1 -> Mux2/3
  Product/1 -> Switch/1
  Abs/1 -> Relay/1
  thetadot_radps2/1 -> Mux2/2
  phidot_radps2/1 -> Mux2/1
  BodyRates_radps/1 -> Mux/1
  Relay/1 -> Switch/2
  Demux/1 -> Mux1/1
  Trigonometric Function/2 -> Demux/1
  EulerAngles_rad/1 -> Trigonometric Function/1
  Mux/1 -> psidot_radps2/1, thetadot_radps2/1, phidot_radps2/1

== system Logan/EqM/EulerAngles/LBE_rotation ==
  note: LBE
  EulerAngles_rad : Inport
  Math Function : Math  Operator=transpose  SignedPower=on
  Mux : Mux  Inputs=2
  Mux2 : Mux  Inputs=9
  Reshape : Reshape  OutputDimensionality=Customize  OutputDimensions=[3,3]
  Trigonometric Function : Trigonometry  Operator=sincos
  phidot_radps1 : Fcn  Expr=u(1)*u(2)*u(6) - u(4)*u(3)
  phidot_radps2 : Fcn  Expr=u(5)*u(6)
  phidot_radps3 : Fcn  Expr=u(6)*u(2)*u(4) + u(1)*u(3)
  phidot_radps4 : Fcn  Expr=u(5)*u(3)
  phidot_radps5 : Fcn  Expr=u(1)*u(2)*u(3) + u(4)*u(6)
  phidot_radps6 : Fcn  Expr=u(4)*u(2)*u(3) -u(1)*u(6)
  phidot_radps7 : Fcn  Expr=-u(2)
  phidot_radps8 : Fcn  Expr=u(1)*u(5)
  phidot_radps9 : Fcn  Expr=u(4)*u(5)
  LBE : Outport
  wires:
  phidot_radps9/1 -> Mux2/9
  phidot_radps8/1 -> Mux2/8
  phidot_radps7/1 -> Mux2/7
  phidot_radps5/1 -> Mux2/5
  phidot_radps6/1 -> Mux2/6
  Mux/1 -> phidot_radps4/1, phidot_radps5/1, phidot_radps6/1, phidot_radps7/1, phidot_radps8/1, phidot_radps9/1, phidot_radps2/1, phidot_radps1/1, phidot_radps3/1
  Trigonometric Function/1 -> Mux/1
  phidot_radps1/1 -> Mux2/2
  phidot_radps2/1 -> Mux2/1
  phidot_radps4/1 -> Mux2/4
  phidot_radps3/1 -> Mux2/3
  Math Function/1 -> LBE/1
  Reshape/1 -> Math Function/1
  Mux2/1 -> Reshape/1
  Trigonometric Function/2 -> Mux/2
  EulerAngles_rad/1 -> Trigonometric Function/1

== system Logan/Inner Loop/LongitudinalControl/GainScheduling1 ==
  Gamma_deg : Inport
  Q_Dyn_Pa : Inport  Port=2
  2-D Lookup Table : Lookup_n-D  NumberOfTableDimensions=1  BreakpointsForDimension1=[83734; 1.70e5; 851500]  BreakpointsForDimension2=[1:3]  Table=[-40; -32; -32]  InternalRulePriority=Speed  RndMeth=Simplest
  Product : Product
  Saturation : Saturate  UpperLimit=-32  LowerLimit=-65
  Out1 : Outport
  wires:
  2-D Lookup Table/1 -> Saturation/1
  Q_Dyn_Pa/1 -> 2-D Lookup Table/1
  Gamma_deg/1 -> Product/1
  Product/1 -> Out1/1
  Saturation/1 -> Product/2

== system Logan/Inner Loop/LongitudinalControl/GainScheduling2 ==
  GammaCmd : Inport
  Q_Dyn_Pa : Inport  Port=2
  2-D Lookup Table : Lookup_n-D  NumberOfTableDimensions=1  BreakpointsForDimension1=[83734; 1.70e5; 851500]  BreakpointsForDimension2=[1:3]  Table=[12; 16;16]  InternalRulePriority=Speed  RndMeth=Simplest
  Product : Product
  Saturation : Saturate  UpperLimit=16  LowerLimit=3
  Out1 : Outport
  wires:
  2-D Lookup Table/1 -> Saturation/1
  Q_Dyn_Pa/1 -> 2-D Lookup Table/1
  GammaCmd/1 -> Product/1
  Product/1 -> Out1/1
  Saturation/1 -> Product/2

== system Logan/Inner Loop/LongitudinalControl/GainScheduling3 ==
  AlphaDot_rps : Inport
  Q_Dyn_Pa : Inport  Port=2
  2-D Lookup Table : Lookup_n-D  NumberOfTableDimensions=1  BreakpointsForDimension1=[83734; 1.70e5; 851500]  BreakpointsForDimension2=[1:3]  Table=[15; 32; 32]  InternalRulePriority=Speed  RndMeth=Simplest
  Product : Product
  Saturation : Saturate  UpperLimit=32  LowerLimit=19
  Out1 : Outport
  wires:
  2-D Lookup Table/1 -> Saturation/1
  Q_Dyn_Pa/1 -> 2-D Lookup Table/1
  AlphaDot_rps/1 -> Product/1
  Product/1 -> Out1/1
  Saturation/1 -> Product/2

== system Logan/Outer Loop/AltitudeMode/Trimming1 ==
  1 : Inport
  Constant17 : Constant  Value=0
  Constant8 : Constant  Value=Trimming
  Switch6 : Switch  Criteria=u2 > Threshold  Threshold=0.5  SaturateOnIntegerOverflow=off  InputSameDT=off
  2 : Outport
  wires:
  Constant8/1 -> Switch6/2
  Constant17/1 -> Switch6/1
  1/1 -> Switch6/3
  Switch6/1 -> 2/1

== system Logan/Outer Loop/BankMode/Trimming1 ==
  1 : Inport
  Constant17 : Constant  Value=0
  Constant8 : Constant  Value=Trimming
  Switch6 : Switch  Criteria=u2 > Threshold  Threshold=0.5  SaturateOnIntegerOverflow=off  InputSameDT=off
  2 : Outport
  wires:
  Constant8/1 -> Switch6/2
  Constant17/1 -> Switch6/1
  1/1 -> Switch6/3
  Switch6/1 -> 2/1

== system Logan/Outer Loop/HeadingMode/Trimming1 ==
  1 : Inport
  Constant17 : Constant  Value=0
  Constant8 : Constant  Value=Trimming
  Switch6 : Switch  Criteria=u2 > Threshold  Threshold=0.5  SaturateOnIntegerOverflow=off  InputSameDT=off
  2 : Outport
  wires:
  Constant8/1 -> Switch6/2
  Constant17/1 -> Switch6/1
  1/1 -> Switch6/3
  Switch6/1 -> 2/1

== system Logan/Outer Loop/TECS/Trimming1 ==
  1 : Inport
  Constant17 : Constant  Value=0
  Constant8 : Constant  Value=Trimming
  Switch6 : Switch  Criteria=u2 > Threshold  Threshold=0.5  SaturateOnIntegerOverflow=off  InputSameDT=off
  2 : Outport
  wires:
  Constant8/1 -> Switch6/2
  Constant17/1 -> Switch6/1
  1/1 -> Switch6/3
  Switch6/1 -> 2/1

== system Logan/Outer Loop/TECS/Trimming2 ==
  1 : Inport
  Constant17 : Constant  Value=0
  Constant8 : Constant  Value=Trimming
  Switch6 : Switch  Criteria=u2 > Threshold  Threshold=0.5  SaturateOnIntegerOverflow=off  InputSameDT=off
  2 : Outport
  wires:
  Constant8/1 -> Switch6/2
  Constant17/1 -> Switch6/1
  1/1 -> Switch6/3
  Switch6/1 -> 2/1

== system Logan/Outer Loop/ThetaMode/Trimming1 ==
  1 : Inport
  Constant17 : Constant  Value=0
  Constant8 : Constant  Value=Trimming
  Switch6 : Switch  Criteria=u2 > Threshold  Threshold=0.5  SaturateOnIntegerOverflow=off  InputSameDT=off
  2 : Outport
  wires:
  Constant8/1 -> Switch6/2
  Constant17/1 -> Switch6/1
  1/1 -> Switch6/3
  Switch6/1 -> 2/1

== system Logan/Propulsion/EngineDynamics/Filter_init ==
  1 : Inport
  Constant : Constant  Value=0
  Constant8 : Constant  Value=Trimming
  Switch6 : Switch  Criteria=u2 > Threshold  Threshold=0.5  SaturateOnIntegerOverflow=off  InputSameDT=off
  2 : Outport
  wires:
  Constant8/1 -> Switch6/2
  Switch6/1 -> 2/1
  1/1 -> Switch6/3
  Constant/1 -> Switch6/1

== system Logan/Propulsion/EngineDynamics/Trimming ==
  Thrust_Dyn : Inport
  Thrust : Inport  Port=2
  Constant8 : Constant  Value=Trimming
  Switch6 : Switch  Criteria=u2 > Threshold  Threshold=0.5  SaturateOnIntegerOverflow=off  InputSameDT=off
  T_Thrust : Outport
  wires:
  Constant8/1 -> Switch6/2
  Switch6/1 -> T_Thrust/1
  Thrust_Dyn/1 -> Switch6/3
  Thrust/1 -> Switch6/1

== system Logan/Propulsion/ScramjetEngine/Ramp_Control ==
  T_Ign : Inport
  T4 : Inport  Port=2
  Add3 : Sum  Inputs=3
  Derivative : Derivative
  First-Order Filter : spsFirstOrderFilterLib/First-Order Filter  FilterType=Lowpass  Tc=30  Ts=0  Initialize=off  Vac_Init=[0, 0, 60]  Vdc_Init=0  PlotResponse=off  FreqRange="[0,  200,  1]"
  Gain : Gain  Gain=5/100
  Gain1 : Gain  Gain=3/100
  Gain2 : Gain  Gain=3/100000
  Gain4 : Gain  Gain=1.10
  Integrator : Integrator  LimitOutput=on  UpperSaturationLimit=10000  LowerSaturationLimit=-10000
  Memory : Memory
  Saturation : Saturate  UpperLimit=14  LowerLimit=-3
  Sum2 : Sum  Inputs=|+-
  Trimming1 : Subsystem
  Trimming2 : Subsystem
  DeltaTheta : Outport
  wires:
  Sum2/1 -> Trimming1/1(1)
  Add3/1 -> Memory/1
  Gain1/1 -> Add3/2
  T_Ign/1 -> Gain4/1
  Integrator/1 -> Gain2/1
  First-Order Filter/1 -> DeltaTheta/1
  Memory/1 -> Saturation/1
  Derivative/1 -> Gain1/1
  Gain2/1 -> Add3/1
  Gain/1 -> Add3/3
  Saturation/1 -> Trimming2/1(1)
  Gain4/1 -> Sum2/1
  T4/1 -> Sum2/2
  Trimming1/1(2) -> Gain/1, Derivative/1, Integrator/1
  Trimming2/1(2) -> First-Order Filter/1

== system Logan/Propulsion/ScramjetEngine/Trimming1 ==
  1 : Inport
  Constant17 : Constant  Value=0
  Constant8 : Constant  Value=Trimming
  Switch6 : Switch  Criteria=u2 > Threshold  Threshold=0.5  SaturateOnIntegerOverflow=off  InputSameDT=off
  2 : Outport
  wires:
  Constant8/1 -> Switch6/2
  Constant17/1 -> Switch6/1
  1/1 -> Switch6/3
  Switch6/1 -> 2/1

== system Logan/Propulsion/ScramjetEngine/Ramp_Control/Trimming1 ==
  1 : Inport
  Constant17 : Constant  Value=0
  Constant8 : Constant  Value=Trimming
  Switch6 : Switch  Criteria=u2 > Threshold  Threshold=0.5  SaturateOnIntegerOverflow=off  InputSameDT=off
  2 : Outport
  wires:
  Constant8/1 -> Switch6/2
  Constant17/1 -> Switch6/1
  1/1 -> Switch6/3
  Switch6/1 -> 2/1

== system Logan/Propulsion/ScramjetEngine/Ramp_Control/Trimming2 ==
  1 : Inport
  Constant17 : Constant  Value=0
  Constant8 : Constant  Value=Trimming
  Switch6 : Switch  Criteria=u2 > Threshold  Threshold=0.5  SaturateOnIntegerOverflow=off  InputSameDT=off
  2 : Outport
  wires:
  Constant8/1 -> Switch6/2
  Constant17/1 -> Switch6/1
  1/1 -> Switch6/3
  Switch6/1 -> 2/1
